simulink model "main_STM32_H743_HIL"  (R2023b)
settings: Solver=FixedStepAuto  StartTime=0.0  StopTime=inf  RelTol=1e-3  EnableMultiTasking=on
values from neighbouring files (symbols this model uses):
  A = 1.87    [parameters.m]
  b_vkm = -10    [parameters.m]
  c_W = 0.4    [parameters.m]
  eta = 0.95    [parameters.m]
  f_R = 0.01    [parameters.m]
  g = 9.81    [parameters.m]
  iD_car = 3.45    [parameters.m]
  iG_car = [0.001 3.682 2.002 1.330 1.000 0.805]    [parameters.m]
  ks_vel = single(3600/(T1_vel*k1_vel*k2_vel))    [parameters.m]
  m_F = 1110    [parameters.m]
  m_vkm = -10/1000    (= -0.01)    [parameters.m]
  m_Zu = 0    [parameters.m]
  p = [-5.1168e-6, 0.0518, 1.1411e+2]    [parameters.m]
  p_L = 1.225    [parameters.m]
  ped_high_deg = 184.57    [parameters.m]
  ped_low_deg = 195.92    [parameters.m]
  ped_m = ped_high_deg - ped_low_deg    (= -11.35)    [parameters.m]
  r_dyn = r_stat    (= 0.30325)    [parameters.m]
  r_stat = (205*0.55*2+15*25.4)/(2*1000)    (= 0.30325)    [parameters.m]
  Ts_acc = 0.1    [parameters.m]
  Ts_ADC = 0.001    [parameters.m]
  UB = 15    [parameters.m]
  v_0 = 130/3.6    (= 36.1111111111)    [parameters.m]
undefined symbols (not defined in the file or in its folder): a_den_vFzg, b_num_vFzg, bits, DiscIntNeverNeededParam
libraries: simulink x14, stm32blockslib x13, stm32h7xxblockslib x7, stm32f4xxblockslib x3, stmutilitieslib x2, dspstat3 x1, svdutilitieslib x1, simulink_extras x1
settings Model: SimulationMode=external  CodeVerificationMode=processor-in-the-loop (pil)  Creator=Sascha  LastModifiedBy=Sascha
settings SolverCC: PositivePriorityOrder=on  AutoInsertRateTranBlk=on
settings DataIOCC: ReturnWorkspaceOutputs=off
settings OptimizationCC: EnhancedBackFolding=on  PassReuseOutputArgsAs=Individual arguments  ZeroExternalMemoryAtStartup=off  ZeroInternalMemoryAtStartup=off  MaxStackSize=64  OptimizeBlockOrder=speed  DifferentSizesBufferReuse=on  OptimizationCustomize=off  EfficientTunableParamExpr=on
settings DebuggingCC: UnderspecifiedInitializationDetection=Classic  MergeDetectMultiDrivingBlocksExec=none  ParameterTunabilityLossMsg=error
settings HardwareCC: ProdBitPerPointer=32  ProdBitPerSizeT=32  ProdBitPerPtrDiffT=32  ProdLargestAtomicInteger=Long  ProdLargestAtomicFloat=Double  ProdWordSize=32  ProdLongLongMode=on  ProdHWDeviceType=ARM Compatible->ARM Cortex
settings SFSimCC: SimCustomHeaderCode="#include \"profile_generator.h\""  SimUserSources=profile_generator.c  SimUserIncludeDirs=..\Modules\  MATLABDynamicMemAlloc=off
settings RTWCC: Description=Embedded Coder  SystemTargetFile=ert.tlc  HardwareBoard=STM32H7xx Based (Single-core)  TemplateMakefile=ert_default_tmf  RTWUseSimCustomCode=on  CustomHeaderCode="#include \"profile_generator.h\""  CustomInclude=..\Modules\  CustomSource=profile_generator.c  Toolchain=GNU Tools for ARM Embedded Processors  CodeExecutionProfiling=on  CodeProfilingSaveOptions=MetricsOnly  CodeProfilingInstrumentation=coarse
settings CodeAppCC: ForceParamTrailComments=on  IgnoreCustomStorageClasses=off  OperatorAnnotations=on  SimulinkDataObjDesc=on  SFDataObjDesc=on  InsertBlockDesc=on
settings ERTTargetCC: TargetLangStandard=C99 (ISO)  CodeReplacementLibrary=ARM Cortex-M  ExtModeTransport=3  ExtModeStaticAlloc=on  ExtModeStaticAllocSize=2048  ExtModeMexFile=ext_xcp  ExtModeIntrfLevel=Level2 - Open

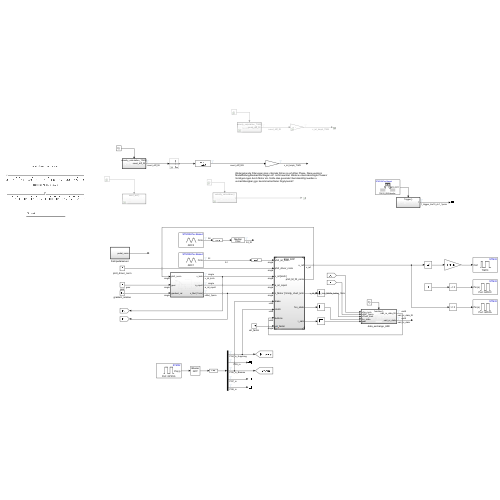
[thumbnail: Simulink's stored preview of the top-level diagram]
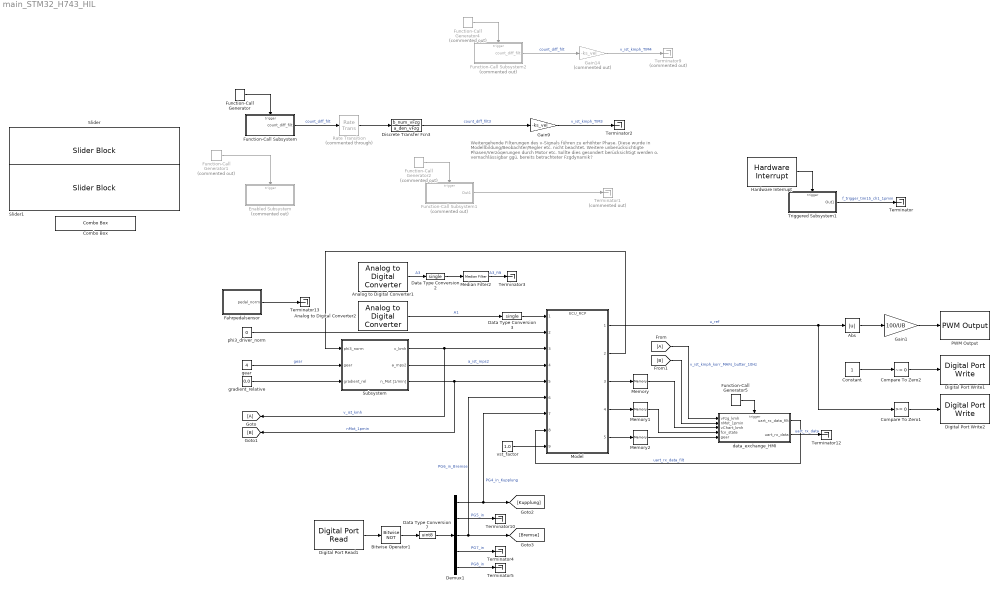
== system main_STM32_H743_HIL ==
  note: Weitergehende Filterungen des v-Signals führen zu erhöhter Phase. Diese wurde in Modellbildung/Beobachter/Regler etc. nicht beachtet. Weitere unberücksichtigte Phasen/Verzögerungen durch Motor etc. Sollte dies gesondert berücksichtigt werden o. vernachlässigbar ggü. bereits betrachteter Fzgdynamik?
  Abs : Abs  SaturateOnIntegerOverflow=off
  Analog to Digital Converter1 : stm32h7xxblockslib/Analog to Digital Converter  ADCModule=ADC3  ConversionGroup=Regular  TriggerMode=Trigger and read  NumberOfConversions=1  EnableBufferConv=off  BufferLength=1  OutputStatus=off  SampleTime=Ts_ADC  EnableSimPort=off
  Analog to Digital Converter2 : stm32h7xxblockslib/Analog to Digital Converter  ADCModule=ADC1  ConversionGroup=Regular  TriggerMode=Trigger and read  NumberOfConversions=1  EnableBufferConv=off  BufferLength=1  OutputStatus=off  SampleTime=Ts_ADC  EnableSimPort=off
  Bitwise Operator1 : simulink/Logic and Bit Operations/Bitwise Operator  logicop=NOT  UseBitMask=off  BitMask=bin2dec('11011001')  BitMaskRealWorld=Stored Integer
  Combo Box : ComboBox  LabelPosition=Hide  SelectedLabel=Gang 4
      settings: Values={{'Approx. Leerlauf', 'Gang 1', 'Gang 2', 'Gang 3', 'Gang 4', 'Gang 5'}, [0 1 2 3 4 5]}
  Compare To Zero1 : simulink/Logic and Bit Operations/Compare To Zero  relop=>=  OutDataTypeStr=boolean
  Compare To Zero2 : simulink/Logic and Bit Operations/Compare To Zero  relop=~=  OutDataTypeStr=boolean
  Constant : Constant
  Data Type Conversion2 : DataTypeConversion  OutDataTypeStr=single  SaturateOnIntegerOverflow=off  RndMeth=Floor
  Data Type Conversion3 : DataTypeConversion  OutDataTypeStr=single  SaturateOnIntegerOverflow=off  RndMeth=Floor
  Data Type Conversion7 : DataTypeConversion  OutDataTypeStr=uint8  SaturateOnIntegerOverflow=off  RndMeth=Floor
  Demux1 : Demux  Outputs=5
  Digital Port Read1 : stm32f4xxblockslib/Digital Port Read  PortName=GPIOG  PinNumber=[4, 5, 6, 7, 8]  ReadOperation=on  IOAsArray=on  SampleTime=0.01  EnableSimPort=off
      settings: LibrarySourceBlock=stm32h7xxblockslib/Digital Port Read
  Digital Port Write1 : stm32f4xxblockslib/Digital Port Write  PortName=GPIOC  PinNumber=[6]  ReadOperation=off  IOAsArray=on  EnableSimPort=off
      settings: LibrarySourceBlock=stm32h7xxblockslib/Digital Port Write
  Digital Port Write2 : stm32f4xxblockslib/Digital Port Write  PortName=GPIOA  PinNumber=[10]  ReadOperation=off  IOAsArray=on  EnableSimPort=off
      settings: LibrarySourceBlock=stm32h7xxblockslib/Digital Port Write
  Discrete Transfer Fcn3 : DiscreteTransferFcn  Numerator=b_num_vFzg  Denominator=a_den_vFzg  SampleTime=0.01
  Enabled Subsystem : Subsystem  Commented=on  TreatAsAtomicUnit=on
  Fahrpedalsensor : Subsystem  TreatAsAtomicUnit=on  SystemSampleTime=Ts_acc*0.1
  From : From
  Function-Call Generator : simulink/Ports & Subsystems/Function-Call Generator  sample_time=T1_vel  numberOfIterations=1  DisallowWideOutput=off
  Function-Call Generator1 : simulink/Ports & Subsystems/Function-Call Generator  Commented=on  sample_time=0.1  numberOfIterations=1  DisallowWideOutput=off
  Function-Call Generator2 : simulink/Ports & Subsystems/Function-Call Generator  Commented=on  sample_time=T1_vel  numberOfIterations=1  DisallowWideOutput=off
  Function-Call Generator4 : simulink/Ports & Subsystems/Function-Call Generator  Commented=on  sample_time=T1_vel  numberOfIterations=1  DisallowWideOutput=off
  Function-Call Generator5 : simulink/Ports & Subsystems/Function-Call Generator  sample_time=0.05  numberOfIterations=1  DisallowWideOutput=off
  Function-Call Subsystem : Subsystem  TreatAsAtomicUnit=on
  Function-Call Subsystem1 : Subsystem  Commented=on  TreatAsAtomicUnit=on
  Function-Call Subsystem2 : Subsystem  Commented=on  TreatAsAtomicUnit=on
  Gain1 : Gain  Gain=100/UB
  Gain14 : Gain  Commented=on  Gain=-ks_vel
  Gain9 : Gain  Gain=-ks_vel
  Goto : Goto
  Hardware Interrupt : stm32h7xxblockslib/Hardware Interrupt  ISRGroup=Timer (TIM)  ISRName=TIM15_IRQHandler  ISRNumber=131  EventsList={ 'off', 'TIM15 Update', '1'; 'on', 'TIM15 CC1', '2'; 'off', 'TIM15 CC2', '3'; 'off', 'TIM15 Trigger', '4'; 'off', 'TIM15 Break', '5'; 'off', 'TIM15 System Break', '6'; 'off', 'TIM15 COM', '7'; 'off', 'Custom event', '8' }  SelectedEvents={'TIM15 CC1'}  TaskPriority=30  DisablePreemption=off  ClearInterruptFlagsAtEndOfEvent=off  InterruptDefinitionFile=$(TARGET_ROOT)/registry/interrupts/STM32F4xxBased_interrupts.xml  HardwareBoard=STM32H7xx Based  EnableSimPort=off
  Median Filter2 : dspstat3/Median Filter  WindowLength=10  SimulateUsing=Code generation
  Memory : Memory
  Memory1 : Memory
  Memory2 : Memory
  Model : ModelReference  ModelNameDialog=ECU_RCP.slx  SimulationMode=Normal  ModelReferenceVersion=7.10
  PWM Output : stm32h7xxblockslib/PWM Output  TimerModule=TIM13  DutycycleUnits=Percentage  EnableChannel1=on  EnableChannel2=off  EnableChannel3=off  EnableChannel4=off  EnableChannel5=off  EnableChannel6=off  EnableCounterInput=off  EnableMainOutputInput=off  EnableFrequencyInput=off  SetRCAfterCE=off  OutputDirection=off  OutputMainOutputEnableStatus=off  SampleTime=0.1  EnableSimPort=off  EnableUpdateEvent=off  EnableCaptureCompare1Event=off  EnableCaptureCompare2Event=off  EnableCaptureCompare3Event=off  EnableCaptureCompare4Event=off  EnableTriggerEvent=off  EnableBreakEvent=off  EnableBreakEvent2=off  ProcessorFamily=STM32H7  hoistedMaskSrc=ECSoC/ECSimCodegen/PWM Output
  Rate Transition : RateTransition  Commented=through  Integrity=off  OutPortSampleTime=0.01
  Slider : SliderBlock  ScaleMax=1
  Slider1 : SliderBlock  ScaleMin=-0.3  ScaleMax=0.3
  Subsystem : Subsystem  TreatAsAtomicUnit=on  SystemSampleTime=0.005
  Terminator{,2..5,10,12..13} (8 alike) : Terminator
  Terminator1 : Terminator  Commented=on
  Terminator9 : Terminator  Commented=on
  Triggered Subsystem1 : Subsystem  TreatAsAtomicUnit=on
  data_exchange_HMI : Subsystem
  gear : Constant  Value=4  OutDataTypeStr=single
  gradient_relative : Constant  Value=0.0  OutDataTypeStr=single
  phi3_driver_norm : Constant  Value=0  OutDataTypeStr=single
  vst_factor : Constant  Value=1.0  OutDataTypeStr=single
  wires:
  Analog to Digital Converter1/1 -> Data Type Conversion2/1  "A3"
  Data Type Conversion2/1 -> Median Filter2/1
  Hardware Interrupt/1 -> Triggered Subsystem1/Trigger
  Function-Call Generator/1 -> Function-Call Subsystem/Trigger
  Function-Call Subsystem/1(count_diff_filt) -> Rate Transition/1  "count_diff_filt"
  Gain9/1 -> Terminator2/1  "v_ist_kmph_TIM3"
  Function-Call Generator1/1 -> Enabled Subsystem/Trigger
  Triggered Subsystem1/1(Out1) -> Terminator/1  "f_trigger_tim15_ch1_1pmin"
  gear/1 -> Subsystem/2(gear)  "gear"
  Model/2 -> Subsystem/1(phi3_norm)
  Subsystem/1(v_kmh) -> Goto/1, Model/3  "v_ist_kmh"
  Subsystem/3(n_Mot [1/min]) -> [B], Model/5  "nMot_1pmin"
  Digital Port Read1/1 -> Bitwise Operator1/1
  Demux1/1 -> Model/7, [Kupplung]  "PG4_in_Kupplung"
  Demux1/2 -> Terminator10/1  "PG5_in"
  phi3_driver_norm/1 -> Model/2
  Demux1/4 -> Terminator4/1  "PG7_in"
  Demux1/5 -> Terminator5/1  "PG8_in"
  Demux1/3 -> Model/6, [Bremse]  "PG6_in_Bremse"
  Bitwise Operator1/1 -> Data Type Conversion7/1
  Subsystem/2(a_mps2) -> Model/4  "a_ist_mps2"
  Data Type Conversion7/1 -> Demux1/1
  Function-Call Generator2/1 -> Function-Call Subsystem1/Trigger
  Function-Call Subsystem1/1(Out1) -> Terminator1/1
  Fahrpedalsensor/1(pedal_norm) -> Terminator13/1
  From/1 -> data_exchange_HMI/1(vFzg_kmh)  "v_ist_kmph_korr_MAFs_butter_10Hz"
  Function-Call Generator4/1 -> Function-Call Subsystem2/Trigger
  Gain14/1 -> Terminator9/1  "v_ist_kmph_TIM4"
  Function-Call Subsystem2/1(count_diff_filt) -> Gain14/1  "count_diff_filt"
  Discrete Transfer Fcn3/1 -> Gain9/1  "count_diff_filt3"
  Rate Transition/1 -> Discrete Transfer Fcn3/1
  Model/1 -> Compare To Zero1/1, Abs/1  "u_ref"
  Constant/1 -> Compare To Zero2/1
  Compare To Zero1/1 -> Digital Port Write2/1
  Abs/1 -> Gain1/1
  Compare To Zero2/1 -> Digital Port Write1/1
  Gain1/1 -> PWM Output/1
  Analog to Digital Converter2/1 -> Data Type Conversion3/1  "A1"
  Data Type Conversion3/1 -> Model/1
  Median Filter2/1 -> Terminator3/1  "A3_filt"
  Function-Call Generator5/1 -> data_exchange_HMI/Trigger
  data_exchange_HMI/1(uart_rx_data_filt) -> Model/8  "uart_rx_data_filt"
  [B] -> data_exchange_HMI/2(nMot_1pmin)
  data_exchange_HMI/2(uart_rx_data) -> Terminator12/1  "uart_rx_data"
  Model/3 -> Memory/1
  Memory/1 -> data_exchange_HMI/3(vChart_kmh)
  Model/4 -> Memory1/1
  Memory1/1 -> data_exchange_HMI/4(fcn_state)
  Model/5 -> Memory2/1
  Memory2/1 -> data_exchange_HMI/5(gear)
  gradient_relative/1 -> Subsystem/3(gradient_rel)
  vst_factor/1 -> Model/9

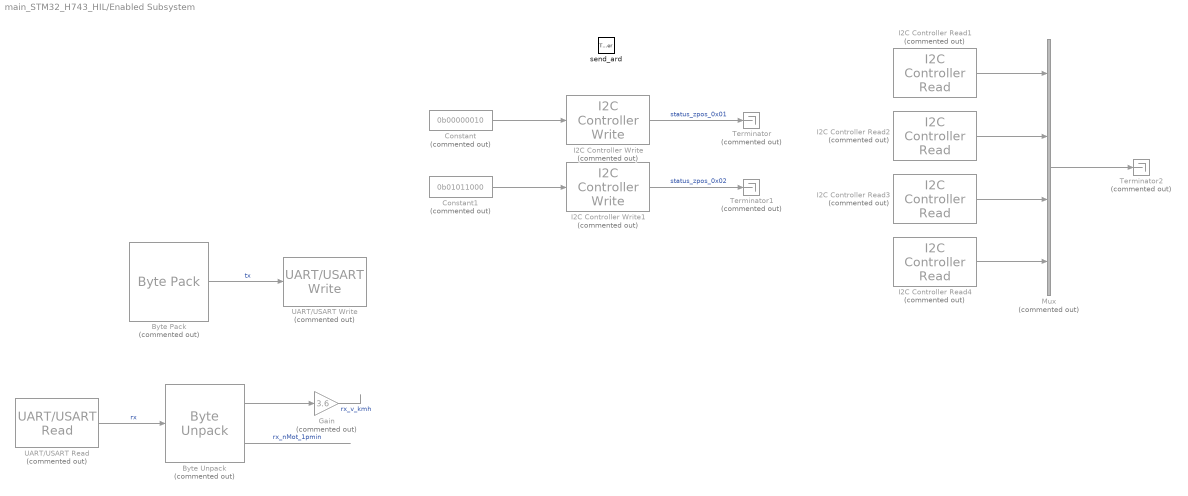
== system main_STM32_H743_HIL/Enabled Subsystem ==
  send_ard : TriggerPort  TriggerType=function-call  VariantControl=(inherit)
  Byte Pack : stmutilitieslib/Byte Pack  Commented=on  datatypes={'single','uint8'}  byteAlign=1  blockPlatform=stm32f4discovery
  Byte Unpack : stmutilitieslib/Byte Unpack  Commented=on  dimensions={[1],[1]}  datatypes={'single','single'}  byteAlign=1  blockPlatform=stm32f4discovery
  Constant : Constant  Commented=on  Value=0b00000010  OutDataTypeStr=uint8
  Constant1 : Constant  Commented=on  Value=0b01011000  OutDataTypeStr=uint8
  Gain : Gain  Commented=on  Gain=3.6
  I2C Controller Read1 : stm32blockslib/I2C Controller Read  Commented=on  I2CModule=I2C1  Mode=Controller  AddressingMode=7-bits  PeripheralByteOrder=BigEndian  OwnPeripheralAddress=uint8(170)  PeripheralAddressVia=Dialog  PeripheralAddress=i2c_addr_acc  RegisterAddressMode=on  RegisterAddressVia=Dialog  RegisterAddress=0x0c  RepeatedStart=off  NoAck=off  OutputStatus=off  BlockMode=Receive  DataType=uint8  DataLength=1  Timeout=i2c_timeout_acc  SampleTime=Ts_acc
      settings: LibrarySourceBlock=stm32f7xxblockslib/I2C Controller Read
  I2C Controller Read2 : stm32blockslib/I2C Controller Read  Commented=on  I2CModule=I2C1  Mode=Controller  AddressingMode=7-bits  PeripheralByteOrder=BigEndian  OwnPeripheralAddress=uint8(170)  PeripheralAddressVia=Dialog  PeripheralAddress=i2c_addr_acc  RegisterAddressMode=on  RegisterAddressVia=Dialog  RegisterAddress=0x0d  RepeatedStart=off  NoAck=off  OutputStatus=off  BlockMode=Receive  DataType=uint8  DataLength=1  Timeout=i2c_timeout_acc  SampleTime=Ts_acc
      settings: LibrarySourceBlock=stm32f7xxblockslib/I2C Controller Read
  I2C Controller Read3 : stm32blockslib/I2C Controller Read  Commented=on  I2CModule=I2C1  Mode=Controller  AddressingMode=7-bits  PeripheralByteOrder=BigEndian  OwnPeripheralAddress=uint8(170)  PeripheralAddressVia=Dialog  PeripheralAddress=i2c_addr_acc  RegisterAddressMode=on  RegisterAddressVia=Dialog  RegisterAddress=0x0e  RepeatedStart=off  NoAck=off  OutputStatus=off  BlockMode=Receive  DataType=uint8  DataLength=1  Timeout=0.001  SampleTime=Ts_acc
      settings: LibrarySourceBlock=stm32f7xxblockslib/I2C Controller Read
  I2C Controller Read4 : stm32blockslib/I2C Controller Read  Commented=on  I2CModule=I2C1  Mode=Controller  AddressingMode=7-bits  PeripheralByteOrder=BigEndian  OwnPeripheralAddress=uint8(170)  PeripheralAddressVia=Dialog  PeripheralAddress=i2c_addr_acc  RegisterAddressMode=on  RegisterAddressVia=Dialog  RegisterAddress=0x0f  RepeatedStart=off  NoAck=off  OutputStatus=off  BlockMode=Receive  DataType=uint8  DataLength=1  Timeout=0.001  SampleTime=Ts_acc
      settings: LibrarySourceBlock=stm32f7xxblockslib/I2C Controller Read
  I2C Controller Write : stm32blockslib/I2C Controller Write  Commented=on  I2CModule=I2C1  Mode=Controller  AddressingMode=7-bits  PeripheralByteOrder=BigEndian  OwnPeripheralAddress=uint8(170)  PeripheralAddressVia=Dialog  PeripheralAddress=i2c_addr_acc  RegisterAddressMode=on  RegisterAddressVia=Dialog  RegisterAddress=0x01  RepeatedStart=off  NoAck=off  OutputStatus=on  BlockMode=Transmit  DataType=uint8  DataLength=1  Timeout=0.001  SampleTime=-1
      settings: LibrarySourceBlock=stm32f7xxblockslib/I2C Controller Write
  I2C Controller Write1 : stm32blockslib/I2C Controller Write  Commented=on  I2CModule=I2C1  Mode=Controller  AddressingMode=7-bits  PeripheralByteOrder=BigEndian  OwnPeripheralAddress=uint8(170)  PeripheralAddressVia=Dialog  PeripheralAddress=i2c_addr_acc  RegisterAddressMode=on  RegisterAddressVia=Dialog  RegisterAddress=0x02  RepeatedStart=off  NoAck=off  OutputStatus=on  BlockMode=Transmit  DataType=uint8  DataLength=1  Timeout=0.001  SampleTime=-1
      settings: LibrarySourceBlock=stm32f7xxblockslib/I2C Controller Write
  Mux : Mux  Commented=on
  Terminator : Terminator  Commented=on
  Terminator1 : Terminator  Commented=on
  Terminator2 : Terminator  Commented=on
  UART/USART Read : stm32blockslib/UART//USART Read  Priority=2  Commented=on  UARTModule=USART6  DataType=uint8  DataLength=8  BlockingMode=off  BlockingTimeout=0.1  OutputLength=off  OutputStatus=off  SampleTime=-1
      settings: LibrarySourceBlock=stm32f7xxblockslib/UART//USART Read
  UART/USART Write : stm32blockslib/UART//USART Write  Priority=1  Commented=on  UARTModule=USART6  LengthOfDataToSend=off  BlockingMode=off  BlockingTimeout=0.1  OutputStatus=off
      settings: LibrarySourceBlock=stm32f7xxblockslib/UART//USART Write
  wires:
  I2C Controller Write/1 -> Terminator/1  "status_zpos_0x01"
  Constant/1 -> I2C Controller Write/1
  Constant1/1 -> I2C Controller Write1/1
  I2C Controller Write1/1 -> Terminator1/1  "status_zpos_0x02"
  I2C Controller Read3/1 -> Mux/3
  I2C Controller Read1/1 -> Mux/1
  I2C Controller Read4/1 -> Mux/4
  Mux/1 -> Terminator2/1
  I2C Controller Read2/1 -> Mux/2
  UART/USART Read/1 -> Byte Unpack/1  "rx"
  Gain/1 -> ?  "rx_v_kmh"
  Byte Pack/1 -> UART/USART Write/1  "tx"
  Byte Unpack/1 -> Gain/1
  Byte Unpack/2 -> ?  "rx_nMot_1pmin"

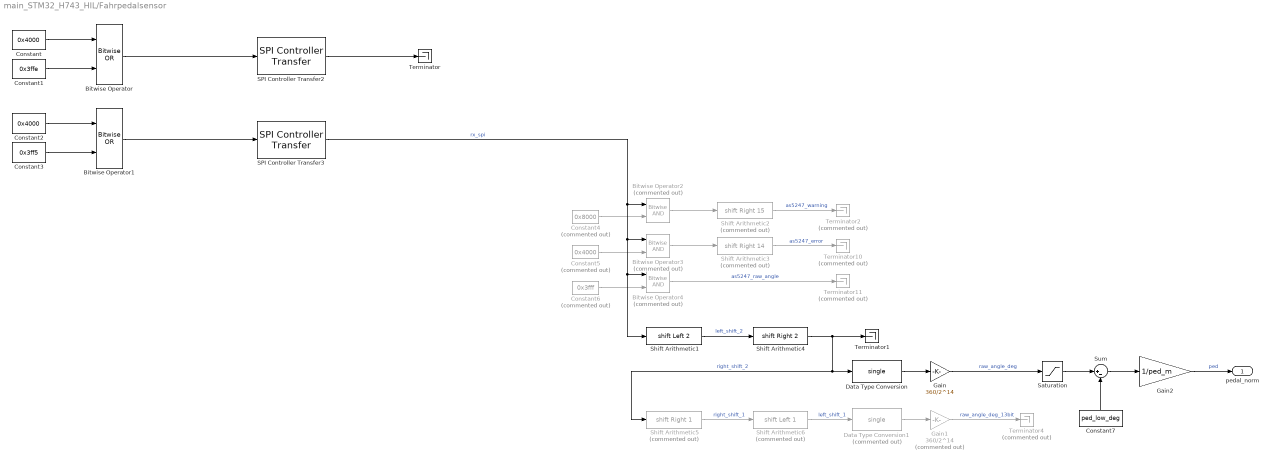
== system main_STM32_H743_HIL/Fahrpedalsensor ==
  Bitwise Operator : simulink/Logic and Bit Operations/Bitwise Operator  logicop=OR  UseBitMask=off  NumInputPorts=2  BitMask=bin2dec('11011001')  BitMaskRealWorld=Stored Integer
  Bitwise Operator1 : simulink/Logic and Bit Operations/Bitwise Operator  logicop=OR  UseBitMask=off  NumInputPorts=2  BitMask=bin2dec('11011001')  BitMaskRealWorld=Stored Integer
  Bitwise Operator2 : simulink/Logic and Bit Operations/Bitwise Operator  Commented=on  logicop=AND  UseBitMask=off  NumInputPorts=2  BitMask=0x8000  BitMaskRealWorld=Stored Integer
  Bitwise Operator3 : simulink/Logic and Bit Operations/Bitwise Operator  Commented=on  logicop=AND  UseBitMask=off  NumInputPorts=2  BitMask=0x4000  BitMaskRealWorld=Stored Integer
  Bitwise Operator4 : simulink/Logic and Bit Operations/Bitwise Operator  Commented=on  logicop=AND  UseBitMask=off  NumInputPorts=2  BitMask=0x3fff  BitMaskRealWorld=Stored Integer
  Constant : Constant  Value=0x4000  OutDataTypeStr=uint16
  Constant1 : Constant  Value=0x3ffe  OutDataTypeStr=uint16
  Constant2 : Constant  Value=0x4000  OutDataTypeStr=uint16
  Constant3 : Constant  Value=0x3ff5  OutDataTypeStr=uint16
  Constant4 : Constant  Commented=on  Value=0x8000  OutDataTypeStr=uint16
  Constant5 : Constant  Commented=on  Value=0x4000  OutDataTypeStr=uint16
  Constant6 : Constant  Commented=on  Value=0x3fff  OutDataTypeStr=uint16
  Constant7 : Constant  Value=ped_low_deg  OutDataTypeStr=single
  Data Type Conversion : DataTypeConversion  OutDataTypeStr=single  SaturateOnIntegerOverflow=off  RndMeth=Floor
  Data Type Conversion1 : DataTypeConversion  Commented=on  OutDataTypeStr=single  SaturateOnIntegerOverflow=off  RndMeth=Floor
  Gain : Gain  Gain=360/2^14
  Gain1 : Gain  Commented=on  Gain=360/2^14
  Gain2 : Gain  Gain=1/ped_m
  SPI Controller Transfer2 : stm32blockslib/SPI Controller Transfer  SPIModuleSelect=SPI3  ClockPolarity=Low  ClockPhase=1 Edge  SPIModule=uint32(0)  Mode=Master  BusSpeed=uint32(1000000)  FirstBitToTransfer=Most significant bit (MSB)  ClockMode=0  BlockFunction=Transfer  EnableRegisterAddress=off  RegisterAddress=0  OutputDataType=uint8  OutputDataLength=1  OutputStatus=off  BlockingMode=off  Timeout=0.001  DataBits=16  UseCustomSSPin=Provided by the SPI peripheral  ActiveLowSSPin=Active low  Port_Select=GPIOA  Pin=0
      settings: LibrarySourceBlock=stm32h7xxblockslib/SPI Controller Transfer
  SPI Controller Transfer3 : stm32blockslib/SPI Controller Transfer  SPIModuleSelect=SPI3  ClockPolarity=Low  ClockPhase=1 Edge  SPIModule=uint32(0)  Mode=Master  BusSpeed=uint32(1000000)  FirstBitToTransfer=Most significant bit (MSB)  ClockMode=0  BlockFunction=Transfer  EnableRegisterAddress=off  RegisterAddress=0  OutputDataType=uint8  OutputDataLength=1  OutputStatus=off  BlockingMode=off  Timeout=0.001  DataBits=16  UseCustomSSPin=Provided by the SPI peripheral  ActiveLowSSPin=Active low  Port_Select=GPIOA  Pin=0
      settings: LibrarySourceBlock=stm32h7xxblockslib/SPI Controller Transfer
  Saturation : Saturate  UpperLimit=ped_low_deg  LowerLimit=ped_high_deg
  Shift Arithmetic1 : ArithShift  BitShiftNumber=2  BitShiftDirection=Left
  Shift Arithmetic2 : ArithShift  Commented=on  BitShiftNumber=15  BitShiftDirection=Right
  Shift Arithmetic3 : ArithShift  Commented=on  BitShiftNumber=14  BitShiftDirection=Right
  Shift Arithmetic4 : ArithShift  BitShiftNumber=2  BitShiftDirection=Right
  Shift Arithmetic5 : ArithShift  Commented=on  BitShiftNumber=1  BitShiftDirection=Right
  Shift Arithmetic6 : ArithShift  Commented=on  BitShiftNumber=1  BitShiftDirection=Left
  Sum : Sum  Inputs=|+-
  Terminator : Terminator
  Terminator1 : Terminator
  Terminator{2,4,10..11} (4 alike) : Terminator  Commented=on
  pedal_norm : Outport
  wires:
  Bitwise Operator/1 -> SPI Controller Transfer2/1
  Constant/1 -> Bitwise Operator/1
  Constant1/1 -> Bitwise Operator/2
  Constant3/1 -> Bitwise Operator1/2
  Constant2/1 -> Bitwise Operator1/1
  Bitwise Operator1/1 -> SPI Controller Transfer3/1
  Constant4/1 -> Bitwise Operator2/2
  Constant5/1 -> Bitwise Operator3/2
  Shift Arithmetic3/1 -> Terminator10/1  "as5247_error"
  Shift Arithmetic2/1 -> Terminator2/1  "as5247_warning"
  Bitwise Operator4/1 -> Terminator11/1  "as5247_raw_angle"
  Bitwise Operator2/1 -> Shift Arithmetic2/1
  Constant6/1 -> Bitwise Operator4/2
  Bitwise Operator3/1 -> Shift Arithmetic3/1
  SPI Controller Transfer3/1 -> Shift Arithmetic1/1, Bitwise Operator4/1, Bitwise Operator3/1, Bitwise Operator2/1  "rx_spi"
  Shift Arithmetic1/1 -> Shift Arithmetic4/1  "left_shift_2"
  Shift Arithmetic4/1 -> Data Type Conversion/1, Shift Arithmetic5/1, Terminator1/1  "right_shift_2"
  Data Type Conversion/1 -> Gain/1
  Gain/1 -> Saturation/1  "raw_angle_deg"
  Shift Arithmetic5/1 -> Shift Arithmetic6/1  "right_shift_1"
  Gain1/1 -> Terminator4/1  "raw_angle_deg_13bit"
  Data Type Conversion1/1 -> Gain1/1
  Shift Arithmetic6/1 -> Data Type Conversion1/1  "left_shift_1"
  SPI Controller Transfer2/1 -> Terminator/1
  Saturation/1 -> Sum/1
  Constant7/1 -> Sum/2
  Sum/1 -> Gain2/1
  Gain2/1 -> pedal_norm/1  "ped"

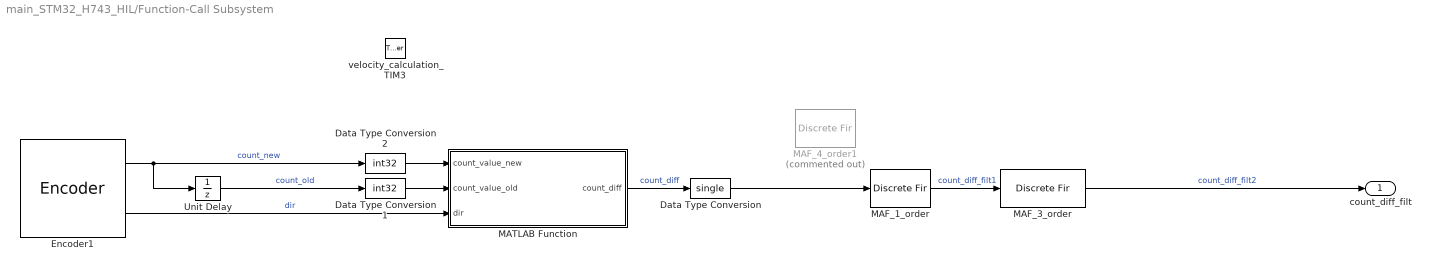
== system main_STM32_H743_HIL/Function-Call Subsystem ==
  velocity_calculation_TIM3 : TriggerPort  TriggerType=function-call  VariantControl=(inherit)
  Data Type Conversion : DataTypeConversion  OutDataTypeStr=single  SaturateOnIntegerOverflow=off  RndMeth=Floor
  Data Type Conversion1 : DataTypeConversion  OutDataTypeStr=int32  SaturateOnIntegerOverflow=off  RndMeth=Floor
  Data Type Conversion2 : DataTypeConversion  OutDataTypeStr=int32  SaturateOnIntegerOverflow=off  RndMeth=Floor
  Encoder1 : stm32blockslib/Encoder  TimerModule=TIM3  EnableResetInput=off  OutputDirection=on  SampleTime=-1
      settings: LibrarySourceBlock=stm32h7xxblockslib/Encoder
  MAF_1_order : DiscreteFir  Coefficients=0.5*[1 1]
  MAF_3_order : DiscreteFir  Coefficients=0.25*[1 1 1 1]
  MAF_4_order1 : DiscreteFir  Commented=on  Coefficients=0.2*[1 1 1 1 1]
  MATLAB Function : MATLAB Function  TreatAsAtomicUnit=on
  Unit Delay : UnitDelay  SampleTime=-1  HasFrameUpgradeWarning=on
  count_diff_filt : Outport
  wires:
  Unit Delay/1 -> Data Type Conversion1/1  "count_old"
  Encoder1/2 -> MATLAB Function/3(dir)  "dir"
  Encoder1/1 -> Unit Delay/1, Data Type Conversion2/1  "count_new"
  MATLAB Function/1(count_diff) -> Data Type Conversion/1  "count_diff"
  Data Type Conversion/1 -> MAF_1_order/1
  Data Type Conversion2/1 -> MATLAB Function/1(count_value_new)
  Data Type Conversion1/1 -> MATLAB Function/2(count_value_old)
  MAF_3_order/1 -> count_diff_filt/1  "count_diff_filt2"
  MAF_1_order/1 -> MAF_3_order/1  "count_diff_filt1"

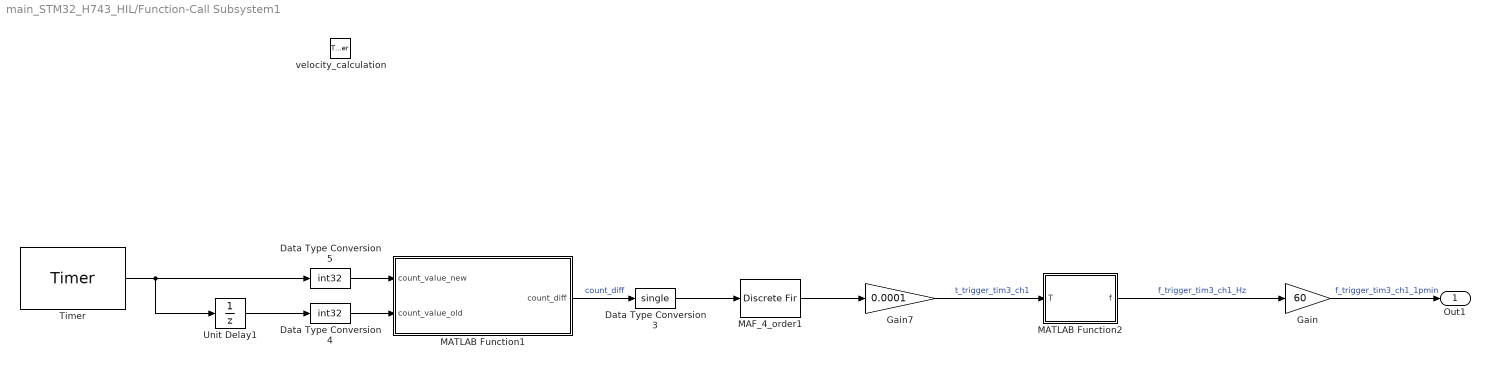
== system main_STM32_H743_HIL/Function-Call Subsystem1 ==
  velocity_calculation : TriggerPort  TriggerType=function-call  VariantControl=(inherit)
  Data Type Conversion3 : DataTypeConversion  OutDataTypeStr=single  SaturateOnIntegerOverflow=off  RndMeth=Floor
  Data Type Conversion4 : DataTypeConversion  OutDataTypeStr=int32  SaturateOnIntegerOverflow=off  RndMeth=Floor
  Data Type Conversion5 : DataTypeConversion  OutDataTypeStr=int32  SaturateOnIntegerOverflow=off  RndMeth=Floor
  Gain : Gain  Gain=60
  Gain7 : Gain  Gain=0.0001
  MAF_4_order1 : DiscreteFir  Coefficients=0.2*[1 1 1 1 1]
  MATLAB Function1 : MATLAB Function  TreatAsAtomicUnit=on
  MATLAB Function2 : MATLAB Function  TreatAsAtomicUnit=on
  Timer : stm32blockslib/Timer  Priority=4  TimerModule=TIM15  EnableFrequencyInput=off  EnableCounterInput=off  EnableMainOutputInput=off  SetRCAfterCE=off  OutputDirection=off  OutputMainOutputEnableStatus=off  SampleTime=-1  EnableUpdateEvent=off  EnableCaptureCompare1Event=off  EnableCaptureCompare2Event=off  EnableCaptureCompare3Event=off  EnableCaptureCompare4Event=off  EnableTriggerEvent=off  EnableBreakEvent=off  EnableBreakEvent2=off  EnableCOMGenerationEvent=off  ProcessorFamily=STM32H7
      settings: LibrarySourceBlock=stm32h7xxblockslib/Timer
  Unit Delay1 : UnitDelay  SampleTime=-1  HasFrameUpgradeWarning=on
  Out1 : Outport
  wires:
  Gain/1 -> Out1/1  "f_trigger_tim3_ch1_1pmin"
  Data Type Conversion5/1 -> MATLAB Function1/1(count_value_new)
  MATLAB Function2/1(f) -> Gain/1  "f_trigger_tim3_ch1_Hz"
  Data Type Conversion4/1 -> MATLAB Function1/2(count_value_old)
  Data Type Conversion3/1 -> MAF_4_order1/1
  Gain7/1 -> MATLAB Function2/1(T)  "t_trigger_tim3_ch1"
  MAF_4_order1/1 -> Gain7/1
  Unit Delay1/1 -> Data Type Conversion4/1
  MATLAB Function1/1(count_diff) -> Data Type Conversion3/1  "count_diff"
  Timer/1 -> Unit Delay1/1, Data Type Conversion5/1

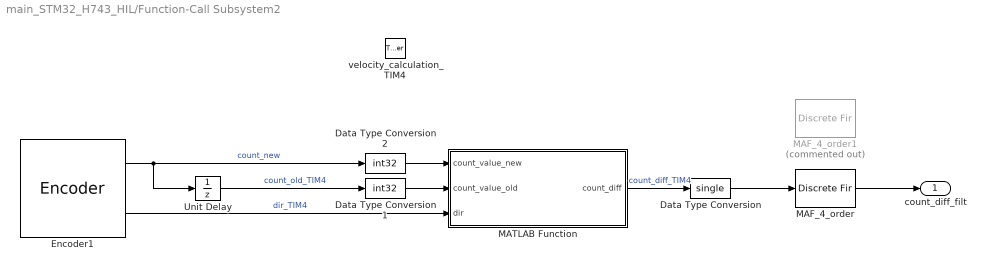
== system main_STM32_H743_HIL/Function-Call Subsystem2 ==
  velocity_calculation_TIM4 : TriggerPort  TriggerType=function-call  VariantControl=(inherit)
  Data Type Conversion : DataTypeConversion  OutDataTypeStr=single  SaturateOnIntegerOverflow=off  RndMeth=Floor
  Data Type Conversion1 : DataTypeConversion  OutDataTypeStr=int32  SaturateOnIntegerOverflow=off  RndMeth=Floor
  Data Type Conversion2 : DataTypeConversion  OutDataTypeStr=int32  SaturateOnIntegerOverflow=off  RndMeth=Floor
  Encoder1 : stm32blockslib/Encoder  TimerModule=TIM4  EnableResetInput=off  OutputDirection=on  SampleTime=-1
      settings: LibrarySourceBlock=stm32h7xxblockslib/Encoder
  MAF_4_order : DiscreteFir  Coefficients=0.5*[1 1]
  MAF_4_order1 : DiscreteFir  Commented=on  Coefficients=0.2*[1 1 1 1 1]
  MATLAB Function : MATLAB Function  TreatAsAtomicUnit=on
  Unit Delay : UnitDelay  SampleTime=-1  HasFrameUpgradeWarning=on
  count_diff_filt : Outport
  wires:
  Unit Delay/1 -> Data Type Conversion1/1  "count_old_TIM4"
  Encoder1/2 -> MATLAB Function/3(dir)  "dir_TIM4"
  Encoder1/1 -> Unit Delay/1, Data Type Conversion2/1  "count_new"
  MATLAB Function/1(count_diff) -> Data Type Conversion/1  "count_diff_TIM4"
  Data Type Conversion/1 -> MAF_4_order/1
  MAF_4_order/1 -> count_diff_filt/1
  Data Type Conversion2/1 -> MATLAB Function/1(count_value_new)
  Data Type Conversion1/1 -> MATLAB Function/2(count_value_old)

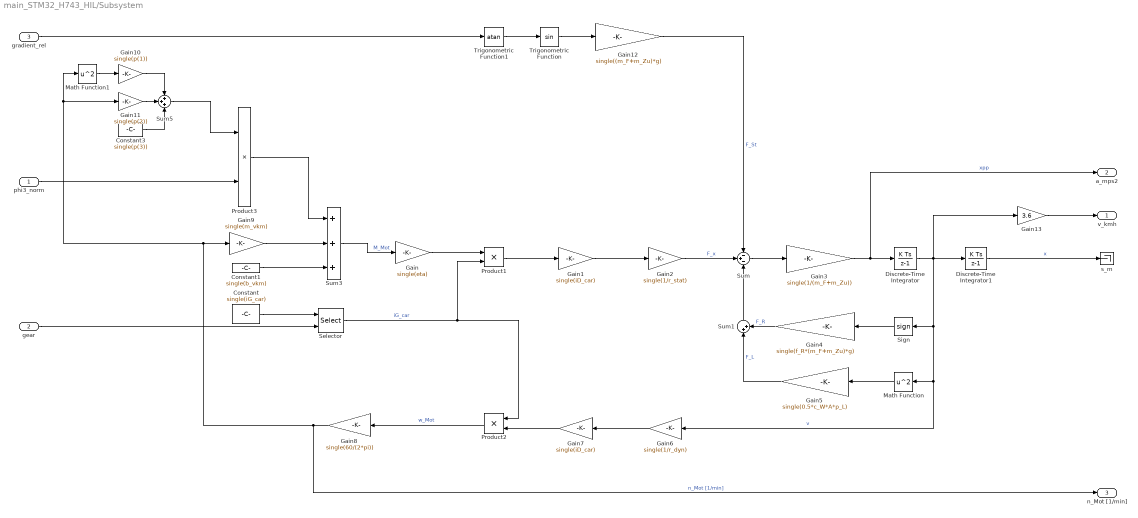
== system main_STM32_H743_HIL/Subsystem ==
  phi3_norm : Inport  OutDataTypeStr=single
  gear : Inport  Port=2  OutDataTypeStr=single
  gradient_rel : Inport  Port=3  OutDataTypeStr=single
  Constant : Constant  Value=single(iG_car)
  Constant1 : Constant  Value=single(b_vkm)
  Constant3 : Constant  Value=single(p(3))
  Discrete-Time Integrator : DiscreteIntegrator  InitialCondition=v_0  SampleTime=-1  ICPrevOutput=DiscIntNeverNeededParam  ICPrevScaledInput=DiscIntNeverNeededParam
  Discrete-Time Integrator1 : DiscreteIntegrator  SampleTime=-1  ICPrevOutput=DiscIntNeverNeededParam  ICPrevScaledInput=DiscIntNeverNeededParam
  Gain : Gain  Gain=single(eta)
  Gain1 : Gain  Gain=single(iD_car)
  Gain10 : Gain  Gain=single(p(1))
  Gain11 : Gain  Gain=single(p(2))
  Gain12 : Gain  Gain=single((m_F+m_Zu)*g)
  Gain13 : Gain  Gain=3.6
  Gain2 : Gain  Gain=single(1/r_stat)
  Gain3 : Gain  Gain=single(1/(m_F+m_Zu))
  Gain4 : Gain  Gain=single(f_R*(m_F+m_Zu)*g)
  Gain5 : Gain  Gain=single(0.5*c_W*A*p_L)
  Gain6 : Gain  Gain=single(1/r_dyn)
  Gain7 : Gain  Gain=single(iD_car)
  Gain8 : Gain  Gain=single(60/(2*pi))
  Gain9 : Gain  Gain=single(m_vkm)
  Math Function : Math  Operator=square
  Math Function1 : Math  Operator=square
  Product1 : Product
  Product2 : Product
  Product3 : Product
  Selector : Selector  IndexMode=Zero-based  InputPortWidth=6  IndexOptions=Index vector (port)  Indices=[1 3]  OutputSizes=1
  Sign : Signum
  Sum : Sum  Inputs=-+-
  Sum1 : Sum  Inputs=|++
  Sum3 : Sum  Inputs=+++
  Sum5 : Sum  Inputs=+++
  Trigonometric Function : Trigonometry
  Trigonometric Function1 : Trigonometry  Operator=atan
  s_m : Terminator
  v_kmh : Outport  OutDataTypeStr=single
  a_mps2 : Outport  Port=2  OutDataTypeStr=single
  n_Mot [1/min] : Outport  Port=3
  wires:
  Gain10/1 -> Sum5/1
  gradient_rel/1 -> Trigonometric Function1/1
  Gain11/1 -> Sum5/2
  phi3_norm/1 -> Product3/2
  Product3/1 -> Sum3/1
  Gain12/1 -> Sum/1  "F_St"
  Gain7/1 -> Product2/2
  Sign/1 -> Gain4/1
  Trigonometric Function1/1 -> Trigonometric Function/1
  Product1/1 -> Gain1/1
  Math Function1/1 -> Gain10/1
  Constant1/1 -> Sum3/3
  Sum5/1 -> Product3/1
  Gain8/1 -> n_Mot [1/min]/1, Math Function1/1, Gain11/1, Gain9/1  "n_Mot [1/min]"
  Discrete-Time Integrator/1 -> Discrete-Time Integrator1/1, Gain13/1, Gain6/1, Math Function/1, Sign/1  "v"
  gear/1 -> Selector/2
  Product2/1 -> Gain8/1  "w_Mot"
  Constant/1 -> Selector/1
  Constant3/1 -> Sum5/3
  Gain6/1 -> Gain7/1
  Gain5/1 -> Sum1/1  "F_L"
  Sum3/1 -> Gain/1  "M_Mot"
  Discrete-Time Integrator1/1 -> s_m/1  "x"
  Sum/1 -> Gain3/1
  Selector/1 -> Product2/1, Product1/2  "iG_car"
  Gain/1 -> Product1/1
  Gain1/1 -> Gain2/1
  Sum1/1 -> Sum/3
  Gain2/1 -> Sum/2  "F_x"
  Gain4/1 -> Sum1/2  "F_R"
  Math Function/1 -> Gain5/1
  Gain9/1 -> Sum3/2
  Gain3/1 -> Discrete-Time Integrator/1, a_mps2/1  "xpp"
  Trigonometric Function/1 -> Gain12/1
  Gain13/1 -> v_kmh/1

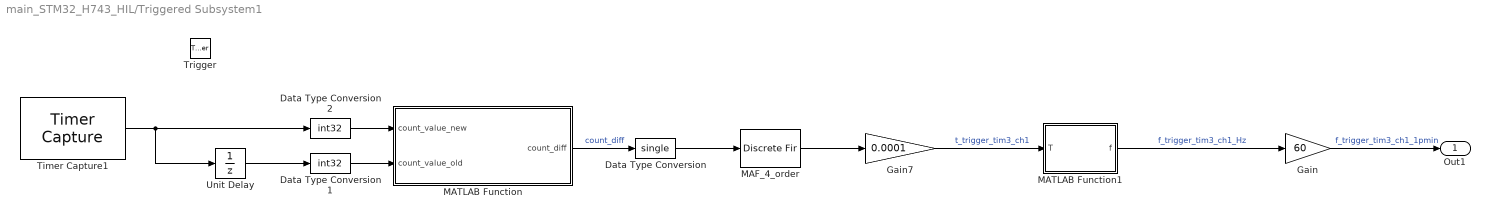
== system main_STM32_H743_HIL/Triggered Subsystem1 ==
  Trigger : TriggerPort  TriggerType=function-call  VariantControl=(inherit)
  Data Type Conversion : DataTypeConversion  OutDataTypeStr=single  SaturateOnIntegerOverflow=off  RndMeth=Floor
  Data Type Conversion1 : DataTypeConversion  OutDataTypeStr=int32  SaturateOnIntegerOverflow=off  RndMeth=Floor
  Data Type Conversion2 : DataTypeConversion  OutDataTypeStr=int32  SaturateOnIntegerOverflow=off  RndMeth=Floor
  Gain : Gain  Gain=60
  Gain7 : Gain  Gain=0.0001
  MAF_4_order : DiscreteFir  Coefficients=0.2*[1 1 1 1 1]
  MATLAB Function : MATLAB Function  TreatAsAtomicUnit=on
  MATLAB Function1 : MATLAB Function  TreatAsAtomicUnit=on
  Timer Capture1 : stm32h7xxblockslib/Timer Capture  TimerModule=TIM15  SelectedChannel=CH1  CaptureLength=1  OutputDataLength=off  OutputOverrunStatus=off  OutputDirection=off  SampleTime=-1
  Unit Delay : UnitDelay  SampleTime=-1  HasFrameUpgradeWarning=on
  Out1 : Outport
  wires:
  Timer Capture1/1 -> Unit Delay/1, Data Type Conversion2/1
  MATLAB Function/1(count_diff) -> Data Type Conversion/1  "count_diff"
  Data Type Conversion/1 -> MAF_4_order/1
  Data Type Conversion2/1 -> MATLAB Function/1(count_value_new)
  Data Type Conversion1/1 -> MATLAB Function/2(count_value_old)
  MAF_4_order/1 -> Gain7/1
  Unit Delay/1 -> Data Type Conversion1/1
  MATLAB Function1/1(f) -> Gain/1  "f_trigger_tim3_ch1_Hz"
  Gain7/1 -> MATLAB Function1/1(T)  "t_trigger_tim3_ch1"
  Gain/1 -> Out1/1  "f_trigger_tim3_ch1_1pmin"

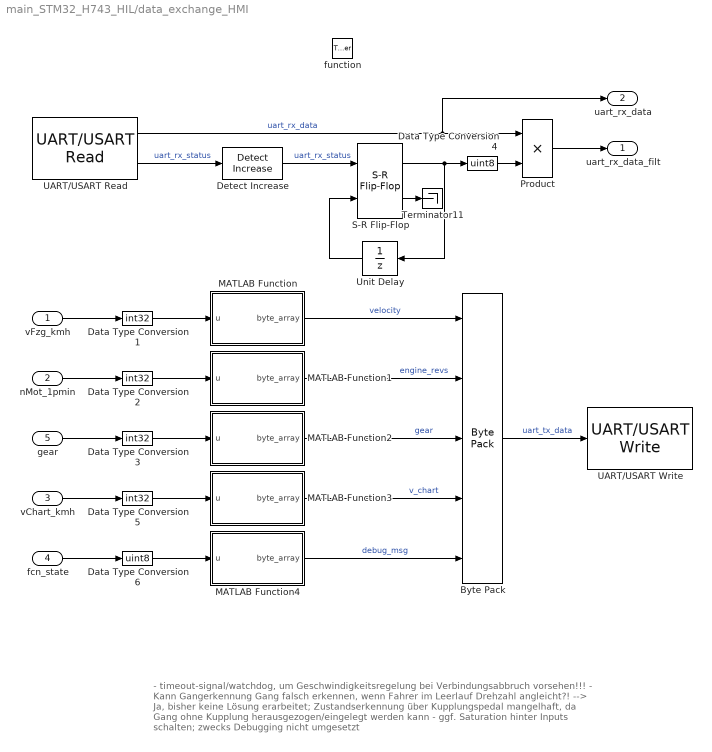
== system main_STM32_H743_HIL/data_exchange_HMI ==
  note: - timeout-signal/watchdog, um Geschwindigkeitsregelung bei Verbindungsabbruch vorsehen!!!
      | - Kann Gangerkennung Gang falsch erkennen, wenn Fahrer im Leerlauf Drehzahl angleicht?! --> Ja, bisher keine Lösung erarbeitet; Zustandserkennung über Kupplungspedal mangelhaft, da Gang ohne Kupplung herausgezogen/eingelegt werden kann
      | - ggf. Saturation hinter Inputs schalten; zwecks Debugging nicht umgesetzt
  vFzg_kmh : Inport
  nMot_1pmin : Inport  Port=2
  vChart_kmh : Inport  Port=3
  fcn_state : Inport  Port=4
  gear : Inport  Port=5
  function : TriggerPort  TriggerType=function-call  VariantControl=(inherit)
  Byte Pack : svdutilitieslib/Byte Pack  maskPackedDataType=uint8  datatypes={'uint8','uint8','uint8','uint8','uint8'}  byteAlign=1  blockPlatform=arduinoert
  Data Type Conversion{1..3,5} (4 alike) : DataTypeConversion  OutDataTypeStr=int32  SaturateOnIntegerOverflow=off  RndMeth=Floor
  Data Type Conversion4 : DataTypeConversion  OutDataTypeStr=uint8  SaturateOnIntegerOverflow=off  RndMeth=Floor
  Data Type Conversion6 : DataTypeConversion  OutDataTypeStr=uint8  SaturateOnIntegerOverflow=off  RndMeth=Floor
  Detect Increase : simulink/Logic and Bit Operations/Detect Increase  vinit=0.0  OutDataTypeStr=boolean
  MATLAB Function : MATLAB Function  TreatAsAtomicUnit=on
  MATLAB Function1 : MATLAB Function  TreatAsAtomicUnit=on
  MATLAB Function2 : MATLAB Function  TreatAsAtomicUnit=on
  MATLAB Function3 : MATLAB Function  TreatAsAtomicUnit=on
  MATLAB Function4 : MATLAB Function  TreatAsAtomicUnit=on
  Product : Product  OutDataTypeStr=uint8
  S-R Flip-Flop : simulink_extras/Flip Flops/S-R Flip-Flop  initial_condition=0
  Terminator11 : Terminator
  UART/USART Read : stm32h7xxblockslib/UART//USART Read  Priority=2  UARTModule=USART2  DataType=uint8  DataLength=1  BlockingMode=off  BlockingTimeout=0.1  OutputLength=off  OutputStatus=on  SampleTime=-1
  UART/USART Write : stm32h7xxblockslib/UART//USART Write  Priority=1  UARTModule=USART2  LengthOfDataToSend=off  BlockingMode=off  BlockingTimeout=0.1  OutputStatus=off
  Unit Delay : UnitDelay  SampleTime=-1  HasFrameUpgradeWarning=on
  uart_rx_data_filt : Outport  OutDataTypeStr=uint8
  uart_rx_data : Outport  Port=2  OutDataTypeStr=uint8
  wires:
  Byte Pack/1 -> UART/USART Write/1  "uart_tx_data"
  MATLAB Function/1(byte_array) -> Byte Pack/1  "velocity"
  MATLAB Function1/1(byte_array) -> Byte Pack/2  "engine_revs"
  MATLAB Function2/1(byte_array) -> Byte Pack/3  "gear"
  Detect Increase/1 -> S-R Flip-Flop/1  "uart_rx_status"
  UART/USART Read/2 -> Detect Increase/1  "uart_rx_status"
  gear/1 -> Data Type Conversion3/1
  nMot_1pmin/1 -> Data Type Conversion2/1
  vFzg_kmh/1 -> Data Type Conversion1/1
  Data Type Conversion1/1 -> MATLAB Function/1(u)
  Data Type Conversion2/1 -> MATLAB Function1/1(u)
  Data Type Conversion3/1 -> MATLAB Function2/1(u)
  UART/USART Read/1 -> uart_rx_data/1, Product/1  "uart_rx_data"
  Data Type Conversion4/1 -> Product/2
  S-R Flip-Flop/2 -> Terminator11/1
  Unit Delay/1 -> S-R Flip-Flop/2
  S-R Flip-Flop/1 -> Unit Delay/1, Data Type Conversion4/1
  Product/1 -> uart_rx_data_filt/1
  Data Type Conversion5/1 -> MATLAB Function3/1(u)
  MATLAB Function3/1(byte_array) -> Byte Pack/4  "v_chart"
  vChart_kmh/1 -> Data Type Conversion5/1
  Data Type Conversion6/1 -> MATLAB Function4/1(u)
  MATLAB Function4/1(byte_array) -> Byte Pack/5  "debug_msg"
  fcn_state/1 -> Data Type Conversion6/1

== matlab function main_STM32_H743_HIL/Triggered Subsystem1/MATLAB Function1 ==
  data: T input single; f output single
function f = time2freq(T)
    if T > 0.0075
        f = 1/T;
    else
        f = single(0);
    end

== matlab function main_STM32_H743_HIL/Function-Call Subsystem/MATLAB Function ==
  data: count_value_new input; count_value_old input; count_diff output int32; dir input; reload_value parameter
function count_diff = fcn(count_value_new, count_value_old, dir, reload_value)

if count_value_new == count_value_old
    count_diff = int32(0);

elseif count_value_new > count_value_old
    if dir == 0
        count_diff = count_value_new - count_value_old;
    else
        count_diff = count_value_new - reload_value - count_value_old - 1;
    end

else
    if dir == 0
        count_diff = count_value_new + reload_value - count_value_old + 1;
    else
        count_diff = count_value_new - count_value_old;
    end

end

== matlab function main_STM32_H743_HIL/Triggered Subsystem1/MATLAB Function ==
  data: count_value_new input; count_value_old input; count_diff output int32
function count_diff = fcn(count_value_new, count_value_old)

if count_value_new == count_value_old
    count_diff = int32(0);

elseif count_value_new > count_value_old
    count_diff = count_value_new - count_value_old;

else
    count_diff = count_value_new + int32(60000) - count_value_old + 1;
end

== matlab function main_STM32_H743_HIL/Function-Call Subsystem1/MATLAB Function1 ==
  data: count_value_new input; count_value_old input; count_diff output int32
function count_diff = fcn(count_value_new, count_value_old)

if count_value_new == count_value_old
    count_diff = int32(0);

elseif count_value_new > count_value_old
    count_diff = count_value_new - count_value_old;

else
    count_diff = count_value_new + int32(10000) - count_value_old + 1;
end

== matlab function main_STM32_H743_HIL/Function-Call Subsystem1/MATLAB Function2 ==
  data: T input single; f output single
function f = time2freq(T)
    if T > 0.0075
        f = 1/T;
    else
        f = single(0);
    end

== matlab function main_STM32_H743_HIL/data_exchange_HMI/MATLAB Function3 ==
  data: u input int32; byte_array output uint8
function byte_array = fcn(u)

dict = uint8([48 49 50 51 52 53 54 55 56 57]); % Zahlen 0-9
blank = uint8(32);
minus = uint8(45);

num_abs = uint8(abs(u));

byte2 = dict((num_abs-mod(num_abs,100))/100+1);
byte3 = dict((mod(num_abs,100)-mod(num_abs,10))/10+1);
byte4 = dict(mod(num_abs,10)+1);

if(num_abs<100)
    byte2 = blank;
end

if(num_abs<10)
    byte3 = blank;
end

if(sign(u) == -1)
    byte1 = minus;
    if(num_abs<100)
        byte1 = blank;
        byte2 = minus;
    end

    if(num_abs<10)
        byte1 = blank;
        byte2 = blank;
        byte3 = minus;
    end
else
    byte1 = blank;
end

byte_array = [byte1, byte2, byte3, byte4];

== matlab function main_STM32_H743_HIL/data_exchange_HMI/MATLAB Function4 ==
  data: u input uint8; byte_array output uint8 size=10
function byte_array = fcn(u)

dict = {uint8('manual    ').', ...  % (0) manual driving
        uint8('active    ').', ...  % (1) velocity control active
        uint8('limiter   ').', ...  % (2) velocity limiter active
        uint8('drvr_ovrrd').', ...  % (3) driver override
        uint8('clutch    ').'};     % (4) clutch pressed

byte_array = dict{u+1};

== matlab function main_STM32_H743_HIL/Function-Call Subsystem2/MATLAB Function ==
  data: count_value_new input; count_value_old input; count_diff output int32; dir input; reload_value parameter
function count_diff = fcn(count_value_new, count_value_old, dir, reload_value)

if count_value_new == count_value_old
    count_diff = int32(0);

elseif count_value_new > count_value_old
    if dir == 0
        count_diff = count_value_new - count_value_old;
    else
        count_diff = count_value_new - reload_value - count_value_old - 1;
    end

else
    if dir == 0
        count_diff = count_value_new + reload_value - count_value_old + 1;
    else
        count_diff = count_value_new - count_value_old;
    end

end

== matlab function main_STM32_H743_HIL/data_exchange_HMI/MATLAB Function ==
  data: u input int32; byte_array output uint8
function byte_array = fcn(u)

dict = uint8([48 49 50 51 52 53 54 55 56 57]); % Zahlen 0-9
blank = uint8(32);
minus = uint8(45);

num_abs = uint8(abs(u));

byte2 = dict((num_abs-mod(num_abs,100))/100+1);
byte3 = dict((mod(num_abs,100)-mod(num_abs,10))/10+1);
byte4 = dict(mod(num_abs,10)+1);

if(num_abs<100)
    byte2 = blank;
end

if(num_abs<10)
    byte3 = blank;
end

if(sign(u) == -1)
    byte1 = minus;
    if(num_abs<100)
        byte1 = blank;
        byte2 = minus;
    end

    if(num_abs<10)
        byte1 = blank;
        byte2 = blank;
        byte3 = minus;
    end
else
    byte1 = blank;
end

byte_array = [byte1, byte2, byte3, byte4];

== matlab function main_STM32_H743_HIL/data_exchange_HMI/MATLAB Function1 ==
  data: u input int32; byte_array output uint8
function byte_array = fcn(u)

num_abs = uint32(abs(u));

dict = uint8([48 49 50 51 52 53 54 55 56 57]); % Zahlen 0-9
blank = uint8(32);

temp1 = mod(num_abs,1000);
byte1 = dict((num_abs-temp1)/1000+1);
temp2 = mod(num_abs,100);
byte2 = dict((temp1-temp2)/100+1);
temp3 = mod(num_abs,10);
byte3 = dict((temp2-temp3)/10+1);
byte4 = dict(temp3+1);

if(num_abs<1000)
    byte1 = blank;
end

if(num_abs<100)
    byte2 = blank;
end

if(num_abs<10)
    byte3 = blank;
end

byte_array = [byte1, byte2, byte3, byte4];

== matlab function main_STM32_H743_HIL/data_exchange_HMI/MATLAB Function2 ==
  data: u input int32; byte_array output uint8
function byte_array = fcn(u)

num_abs = uint32(abs(u));

dict = uint8([48 49 50 51 52 53 54 55 56 57]); % Zahlen 0-9
blank = uint8(32);

temp1 = mod(num_abs,1000);
byte1 = dict((num_abs-temp1)/1000+1);
temp2 = mod(num_abs,100);
byte2 = dict((temp1-temp2)/100+1);
temp3 = mod(num_abs,10);
byte3 = dict((temp2-temp3)/10+1);
byte4 = dict(temp3+1);

if(num_abs<1000)
    byte1 = blank;
end

if(num_abs<100)
    byte2 = blank;
end

if(num_abs<10)
    byte3 = blank;
end

byte_array = [byte1, byte2, byte3, byte4];
